simulink model "TESTENV_VisualLanding"  (R2020a)
settings: Solver=ode1  StartTime=0.0  StopTime=inf  FixedStep=Ts_VisualLanding.Ts_Base  RelTol=1e-3
undefined symbols (not defined in the file or in its folder): eulerd_yaw_pitch_roll, idx, lla, PlaneMode, posNED, Rcl, tcl, velNED
libraries: simulink x1
settings Model: PauseTimes=[308,310,12]  Creator=sl  LastModifiedBy=sl
settings DataIOCC: SaveOutput=off  SaveTime=off
settings OptimizationCC: DefaultParameterBehavior=Inlined  EnhancedBackFolding=on  PassReuseOutputArgsAs=Individual arguments  ZeroExternalMemoryAtStartup=off  ZeroInternalMemoryAtStartup=off  OptimizeBlockOrder=speed  DifferentSizesBufferReuse=on  OptimizationCustomize=off  EfficientTunableParamExpr=on
settings DebuggingCC: InheritedTsInSrcMsg=none  ParameterPrecisionLossMsg=none  ParameterTunabilityLossMsg=error  UnconnectedInputMsg=none  UnconnectedOutputMsg=none  UnconnectedLineMsg=none  SFUnusedDataAndEventsDiag=none
settings HardwareCC: ProdBitPerPointer=32  ProdBitPerSizeT=32  ProdBitPerPtrDiffT=32  ProdLargestAtomicInteger=Long  ProdLargestAtomicFloat=Double  ProdWordSize=32  ProdHWDeviceType=ARM Compatible->ARM Cortex
settings ModelReferenceCC: ModelReferenceNumInstancesAllowed=Single
settings SFSimCC: MATLABDynamicMemAlloc=off
settings RTWCC: SystemTargetFile=ert.tlc  TemplateMakefile=ert_default_tmf  GenerateReport=on  IncludeHyperlinkInReport=on  LaunchReport=on  GenerateTraceInfo=on  GenerateTraceReport=on  GenerateTraceReportSl=on  GenerateTraceReportSf=on  GenerateTraceReportEml=on
settings CodeAppCC: ForceParamTrailComments=on  IgnoreCustomStorageClasses=off  MaxIdLength=48  OperatorAnnotations=on  SimulinkDataObjDesc=on  SFDataObjDesc=on  InsertBlockDesc=on
settings ERTTargetCC: TargetLangStandard=C99 (ISO)  GenerateSampleERTMain=on  CombineOutputUpdateFcns=off  LogVarNameModifier=none  SupportVariableSizeSignals=on  InlinedParameterPlacement=NonHierarchical  ERTCustomFileTemplate=example_file_process.tlc

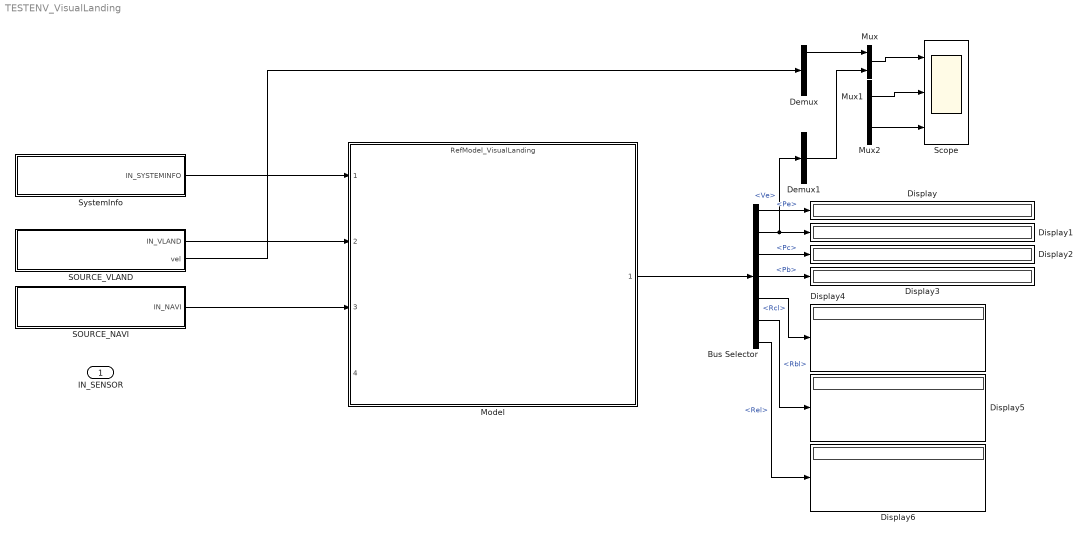
== system TESTENV_VisualLanding ==
  IN_SENSOR : Inport  OutDataTypeStr=Bus: BUS_SENSOR  BusOutputAsStruct=on
  Bus Selector : BusSelector  OutputSignals=Pe,Ve,Pc,Pb,Rcl,Rbl,Rel
  Demux : Demux  Outputs=3
  Demux1 : Demux  Outputs=3
  Display{,1..6} (7 alike) : Display
  Model : ModelReference  ModelNameDialog=RefModel_VisualLanding.slx  SimulationMode=Normal  ModelReferenceVersion=1.2019
  Mux : Mux  Inputs=2
  Mux1 : Mux  Inputs=2
  Mux2 : Mux  Inputs=2
  SOURCE_NAVI : Subsystem
  SOURCE_VLAND : Subsystem
  Scope : Scope  NumInputPorts=3
  SystemInfo : Subsystem
  wires:
  SystemInfo/1(IN_SYSTEMINFO) -> Model/1
  SOURCE_VLAND/1(IN_VLAND) -> Model/2
  SOURCE_NAVI/1(IN_NAVI) -> Model/3
  Model/1 -> Bus Selector/1
  Bus Selector/1 -> Display/1  "<Pe>"
  Bus Selector/2 -> Demux1/1, Display1/1  "<Ve>"
  Bus Selector/3 -> Display2/1  "<Pc>"
  Bus Selector/4 -> Display3/1  "<Pb>"
  Bus Selector/5 -> Display4/1  "<Rcl>"
  Bus Selector/6 -> Display5/1  "<Rbl>"
  Bus Selector/7 -> Display6/1  "<Rel>"
  Demux/1 -> Mux/1
  Mux2/1 -> Scope/3
  Mux/1 -> Scope/1
  Mux1/1 -> Scope/2
  SOURCE_VLAND/2(vel) -> Demux/1
  Demux1/2 -> Mux/2

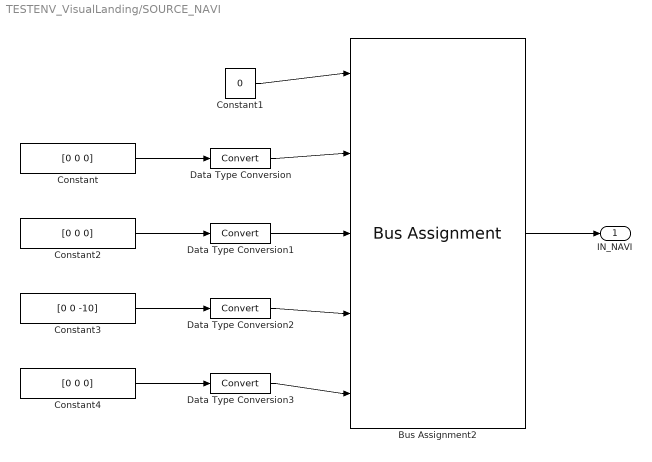
== system TESTENV_VisualLanding/SOURCE_NAVI ==
  Bus Assignment2 : BusAssignment  AssignedSignals=lla,eulerd_yaw_pitch_roll,posNED,velNED
  Constant : Constant  Value=[0 0 0]
  Constant1 : Constant  Value=0  OutDataTypeStr=Bus: BUS_NAVI_TO_FIRM
  Constant2 : Constant  Value=[0 0 0]
  Constant3 : Constant  Value=[0 0 -10]
  Constant4 : Constant  Value=[0 0 0]
  Data Type Conversion{,1..3} (4 alike) : DataTypeConversion
  IN_NAVI : Outport  BusOutputAsStruct=on
  wires:
  Constant/1 -> Data Type Conversion/1
  Constant1/1 -> Bus Assignment2/1
  Bus Assignment2/1 -> IN_NAVI/1
  Constant2/1 -> Data Type Conversion1/1
  Data Type Conversion/1 -> Bus Assignment2/2
  Data Type Conversion1/1 -> Bus Assignment2/3
  Constant3/1 -> Data Type Conversion2/1
  Data Type Conversion2/1 -> Bus Assignment2/4
  Constant4/1 -> Data Type Conversion3/1
  Data Type Conversion3/1 -> Bus Assignment2/5

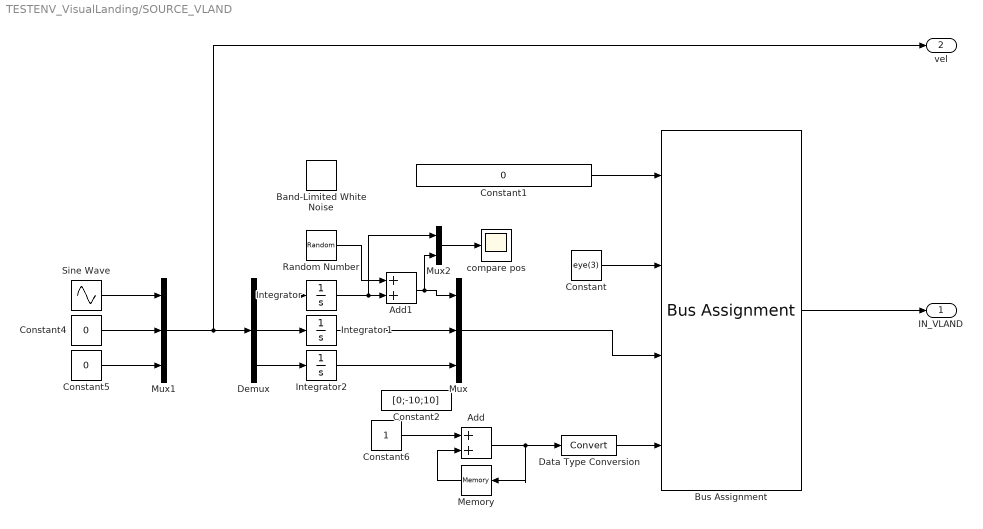
== system TESTENV_VisualLanding/SOURCE_VLAND ==
  Add : Sum
  Add1 : Sum
  Band-Limited White Noise : simulink/Sources/Band-Limited White Noise  Cov=[0.1]  Ts=0.012  seed=[23341]
  Bus Assignment : BusAssignment  AssignedSignals=Rcl,tcl,idx
  Constant : Constant  Value=eye(3)
  Constant1 : Constant  Value=0  OutDataTypeStr=Bus: BUS_VISUALLANDING_INPUT
  Constant2 : Constant  Value=[0;-10;10]
  Constant4 : Constant  Value=0
  Constant5 : Constant  Value=0
  Constant6 : Constant
  Data Type Conversion : DataTypeConversion
  Demux : Demux  Outputs=3
  Integrator : Integrator
  Integrator1 : Integrator
  Integrator2 : Integrator
  Memory : Memory
  Mux : Mux  Inputs=3
  Mux1 : Mux  Inputs=3
  Mux2 : Mux  Inputs=2
  Random Number : RandomNumber
  Sine Wave : Sin  Amplitude=3  Bias=10  Frequency=0.1  SampleTime=0
  compare pos : Scope
  IN_VLAND : Outport
  vel : Outport  Port=2
  wires:
  Bus Assignment/1 -> IN_VLAND/1
  Constant1/1 -> Bus Assignment/1
  Constant/1 -> Bus Assignment/2
  Mux/1 -> Bus Assignment/3
  Demux/1 -> Integrator/1
  Demux/2 -> Integrator1/1
  Integrator1/1 -> Mux/2
  Integrator2/1 -> Mux/3
  Demux/3 -> Integrator2/1
  Constant6/1 -> Add/1
  Add/1 -> Memory/1, Data Type Conversion/1
  Memory/1 -> Add/2
  Data Type Conversion/1 -> Bus Assignment/4
  Sine Wave/1 -> Mux1/1
  Constant4/1 -> Mux1/2
  Constant5/1 -> Mux1/3
  Mux1/1 -> vel/1, Demux/1
  Integrator/1 -> Mux2/1, Add1/2
  Add1/1 -> Mux2/2, Mux/1
  Random Number/1 -> Add1/1
  Mux2/1 -> compare pos/1

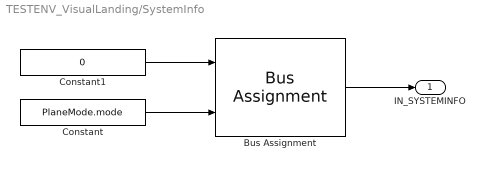
== system TESTENV_VisualLanding/SystemInfo ==
  Bus Assignment : BusAssignment  AssignedSignals=plane_model_control
  Constant : Constant  Value=PlaneMode.mode  OutDataTypeStr=Enum: ENUM_plane_mode
  Constant1 : Constant  Value=0  OutDataTypeStr=Bus: BUS_SYSTEMINFO_INPUT
  IN_SYSTEMINFO : Outport
  wires:
  Constant1/1 -> Bus Assignment/1
  Constant/1 -> Bus Assignment/2
  Bus Assignment/1 -> IN_SYSTEMINFO/1
